simulink model "TCS5"  (R2018b)
settings: Solver=VariableStepAuto  StartTime=0.0  StopTime=10  RelTol=1e-3
model workspace (MAT data in the model file):
  MCOS : class17 (value not decoded)
  MCOS : class17 (value not decoded)
  MCOS : class17 (value not decoded)
  MCOS : class17 (value not decoded)
  MCOS : class17 (value not decoded)
  MCOS : class17 (value not decoded)
undefined symbols (not defined in the file): DiscIntNeverNeededParam
libraries: simulink x8, Solver_SF x1
(part 2 of 2)

== system TCS5/TCS_Control/Axle_3/PID控制器2 ==
  期望驱动力矩 : Inport
  差值 : Inport  Port=2
  Enable : Inport  Port=3
  Abs : Abs
  Add : Sum
  Add1 : Sum
  Constant : Constant  Value=0  OutDataTypeStr=fixdt(1,16,5)
  Constant1 : Constant  Value=T_max
  Constant2 : Constant  Value=Kp
  Constant3 : Constant  Value=Ki
  Constant4 : Constant  Value=0
  Discrete-Time Integrator : DiscreteIntegrator  IntegratorMethod=Integration: Backward Euler  ExternalReset=level  SampleTime=-1  ICPrevOutput=DiscIntNeverNeededParam  ICPrevScaledInput=DiscIntNeverNeededParam
  Logical Operator1 : Logic  Operator=NOT  AllPortsSameDT=off  OutDataTypeStr=boolean
  Multiply : Product  OutDataTypeStr=fixdt(1,32,10)
  Multiply1 : Product  OutDataTypeStr=fixdt(1,32,10)
  Relational Operator : RelationalOperator  Operator===  OutDataTypeStr=boolean  RndMeth=Nearest
  Saturation Dynamic : simulink/Discontinuities/Saturation Dynamic  OutMin=[]  OutMax=[]  OutDataTypeStr=Inherit: Same as second input  OutDataType=fixdt(1, 16)  OutScaling=2^-10  DoSatur=off
  Switch : Switch  Criteria=u2 > Threshold
  Unit Delay : UnitDelay  SampleTime=-1
  △T : Outport  VectorParamsAs1DForOutWhenUnconnected=on
  wires:
  Multiply/1 -> Add/1
  Discrete-Time Integrator/1 -> Add/2
  Enable/1 -> Logical Operator1/1
  Multiply1/1 -> Discrete-Time Integrator/1
  Constant3/1 -> Multiply1/2
  Relational Operator/1 -> Unit Delay/1
  Saturation Dynamic/1 -> Relational Operator/2, △T/1
  Constant2/1 -> Multiply/1
  Unit Delay/1 -> Switch/2
  差值/1 -> Switch/1, Multiply/2
  Add/1 -> Saturation Dynamic/2, Relational Operator/1
  Logical Operator1/1 -> Discrete-Time Integrator/2
  Switch/1 -> Multiply1/1
  Constant/1 -> Switch/3
  Constant1/1 -> Add1/1
  Add1/1 -> Saturation Dynamic/1
  期望驱动力矩/1 -> Abs/1
  Abs/1 -> Add1/2
  Constant4/1 -> Saturation Dynamic/3

== system TCS5/TCS_Control/Axle_3/滑转率计算1 ==
  车轮转速 : Inport
  车速 : Inport  Port=2
  Abs : Abs
  Add : Sum  Inputs=+-
  Add1 : Sum
  Constant : Constant  Value=0.001
  Divide : Product  Inputs=*/
  Gain : Gain  Gain=1/3.6
  Gain2 : Gain  Gain=pi/30
  Product : Product
  Saturation : Saturate  UpperLimit=1  LowerLimit=-1
  轮胎滚动半径 : Constant  Value=r
  左轮滑转率 : Outport  VectorParamsAs1DForOutWhenUnconnected=on
  wires:
  Saturation/1 -> 左轮滑转率/1
  Divide/1 -> Saturation/1
  轮胎滚动半径/1 -> Product/2
  Add/1 -> Divide/1
  Product/1 -> Abs/1, Add/1
  车速/1 -> Gain/1
  Gain/1 -> Add/2
  Gain2/1 -> Product/1
  车轮转速/1 -> Gain2/1
  Add1/1 -> Divide/2
  Constant/1 -> Add1/2
  Abs/1 -> Add1/1

== system TCS5/TCS_Control/Axle_3/滑转率计算2 ==
  车轮转速 : Inport
  车速 : Inport  Port=2
  Abs : Abs
  Add : Sum  Inputs=+-
  Add1 : Sum
  Constant : Constant  Value=0.001
  Divide : Product  Inputs=*/
  Gain : Gain  Gain=1/3.6
  Gain2 : Gain  Gain=pi/30
  Product : Product
  Saturation : Saturate  UpperLimit=1  LowerLimit=-1
  轮胎滚动半径 : Constant  Value=r
  右轮滑转率 : Outport  VectorParamsAs1DForOutWhenUnconnected=on
  wires:
  Saturation/1 -> 右轮滑转率/1
  Divide/1 -> Saturation/1
  轮胎滚动半径/1 -> Product/2
  Add/1 -> Divide/1
  Product/1 -> Abs/1, Add/1
  车速/1 -> Gain/1
  Gain/1 -> Add/2
  Gain2/1 -> Product/1
  车轮转速/1 -> Gain2/1
  Add1/1 -> Divide/2
  Constant/1 -> Add1/2
  Abs/1 -> Add1/1

== system TCS5/TCS_Control/Axle_5/PID控制器1 ==
  期望驱动力矩 : Inport
  差值 : Inport  Port=2
  Enable : Inport  Port=3
  Abs : Abs
  Add : Sum
  Add1 : Sum
  Constant : Constant  Value=0  OutDataTypeStr=fixdt(1,16,5)
  Constant1 : Constant  Value=T_max
  Constant2 : Constant  Value=Kp
  Constant3 : Constant  Value=Ki
  Constant4 : Constant  Value=0
  Discrete-Time Integrator : DiscreteIntegrator  IntegratorMethod=Integration: Backward Euler  ExternalReset=level  SampleTime=-1  ICPrevOutput=DiscIntNeverNeededParam  ICPrevScaledInput=DiscIntNeverNeededParam
  Logical Operator1 : Logic  Operator=NOT  AllPortsSameDT=off  OutDataTypeStr=boolean
  Multiply : Product  OutDataTypeStr=fixdt(1,32,10)
  Multiply1 : Product  OutDataTypeStr=fixdt(1,32,10)
  Relational Operator : RelationalOperator  Operator===  OutDataTypeStr=boolean  RndMeth=Nearest
  Saturation Dynamic : simulink/Discontinuities/Saturation Dynamic  OutMin=[]  OutMax=[]  OutDataTypeStr=Inherit: Same as second input  OutDataType=fixdt(1, 16)  OutScaling=2^-10  DoSatur=off
  Scope : Scope
  Switch : Switch  Criteria=u2 > Threshold
  Unit Delay : UnitDelay  SampleTime=-1
  △T : Outport  VectorParamsAs1DForOutWhenUnconnected=on
  wires:
  Multiply/1 -> Add/1
  Enable/1 -> Logical Operator1/1
  Multiply1/1 -> Discrete-Time Integrator/1
  Constant3/1 -> Multiply1/2
  Relational Operator/1 -> Unit Delay/1
  Saturation Dynamic/1 -> Relational Operator/2, △T/1
  Constant2/1 -> Multiply/1
  Unit Delay/1 -> Switch/2
  差值/1 -> Switch/1, Multiply/2
  Add/1 -> Saturation Dynamic/2, Relational Operator/1
  Logical Operator1/1 -> Discrete-Time Integrator/2
  Switch/1 -> Multiply1/1
  Constant/1 -> Switch/3
  Constant1/1 -> Add1/1
  Add1/1 -> Saturation Dynamic/1
  期望驱动力矩/1 -> Abs/1
  Abs/1 -> Add1/2
  Constant4/1 -> Saturation Dynamic/3
  Discrete-Time Integrator/1 -> Scope/1, Add/2

== system TCS5/TCS_Control/Axle_5/PID控制器2 ==
  期望驱动力矩 : Inport
  差值 : Inport  Port=2
  Enable : Inport  Port=3
  Abs : Abs
  Add : Sum
  Add1 : Sum
  Constant : Constant  Value=0  OutDataTypeStr=fixdt(1,16,5)
  Constant1 : Constant  Value=T_max
  Constant2 : Constant  Value=Kp
  Constant3 : Constant  Value=Ki
  Constant4 : Constant  Value=0
  Discrete-Time Integrator : DiscreteIntegrator  IntegratorMethod=Integration: Backward Euler  ExternalReset=level  SampleTime=-1  ICPrevOutput=DiscIntNeverNeededParam  ICPrevScaledInput=DiscIntNeverNeededParam
  Logical Operator1 : Logic  Operator=NOT  AllPortsSameDT=off  OutDataTypeStr=boolean
  Multiply : Product  OutDataTypeStr=fixdt(1,32,10)
  Multiply1 : Product  OutDataTypeStr=fixdt(1,32,10)
  Relational Operator : RelationalOperator  Operator===  OutDataTypeStr=boolean  RndMeth=Nearest
  Saturation Dynamic : simulink/Discontinuities/Saturation Dynamic  OutMin=[]  OutMax=[]  OutDataTypeStr=Inherit: Same as second input  OutDataType=fixdt(1, 16)  OutScaling=2^-10  DoSatur=off
  Switch : Switch  Criteria=u2 > Threshold
  Unit Delay : UnitDelay  SampleTime=-1
  △T : Outport  VectorParamsAs1DForOutWhenUnconnected=on
  wires:
  Multiply/1 -> Add/1
  Discrete-Time Integrator/1 -> Add/2
  Enable/1 -> Logical Operator1/1
  Multiply1/1 -> Discrete-Time Integrator/1
  Constant3/1 -> Multiply1/2
  Relational Operator/1 -> Unit Delay/1
  Saturation Dynamic/1 -> Relational Operator/2, △T/1
  Constant2/1 -> Multiply/1
  Unit Delay/1 -> Switch/2
  差值/1 -> Switch/1, Multiply/2
  Add/1 -> Saturation Dynamic/2, Relational Operator/1
  Logical Operator1/1 -> Discrete-Time Integrator/2
  Switch/1 -> Multiply1/1
  Constant/1 -> Switch/3
  Constant1/1 -> Add1/1
  Add1/1 -> Saturation Dynamic/1
  期望驱动力矩/1 -> Abs/1
  Abs/1 -> Add1/2
  Constant4/1 -> Saturation Dynamic/3

== system TCS5/TCS_Control/Axle_5/滑转率计算1 ==
  车轮转速 : Inport
  车速 : Inport  Port=2
  Abs : Abs
  Add : Sum  Inputs=+-
  Add1 : Sum
  Constant : Constant  Value=0.001
  Divide : Product  Inputs=*/
  Gain : Gain  Gain=1/3.6
  Gain2 : Gain  Gain=pi/30
  Product : Product
  Saturation : Saturate  UpperLimit=1  LowerLimit=-1
  轮胎滚动半径 : Constant  Value=r
  左轮滑转率 : Outport  VectorParamsAs1DForOutWhenUnconnected=on
  wires:
  Saturation/1 -> 左轮滑转率/1
  Divide/1 -> Saturation/1
  轮胎滚动半径/1 -> Product/2
  Add/1 -> Divide/1
  Product/1 -> Abs/1, Add/1
  车速/1 -> Gain/1
  Gain/1 -> Add/2
  Gain2/1 -> Product/1
  车轮转速/1 -> Gain2/1
  Add1/1 -> Divide/2
  Constant/1 -> Add1/2
  Abs/1 -> Add1/1

== system TCS5/TCS_Control/Axle_5/滑转率计算2 ==
  车轮转速 : Inport
  车速 : Inport  Port=2
  Abs : Abs
  Add : Sum  Inputs=+-
  Add1 : Sum
  Constant : Constant  Value=0.001
  Divide : Product  Inputs=*/
  Gain : Gain  Gain=1/3.6
  Gain2 : Gain  Gain=pi/30
  Product : Product
  Saturation : Saturate  UpperLimit=1  LowerLimit=-1
  轮胎滚动半径 : Constant  Value=r
  右轮滑转率 : Outport  VectorParamsAs1DForOutWhenUnconnected=on
  wires:
  Saturation/1 -> 右轮滑转率/1
  Divide/1 -> Saturation/1
  轮胎滚动半径/1 -> Product/2
  Add/1 -> Divide/1
  Product/1 -> Abs/1, Add/1
  车速/1 -> Gain/1
  Gain/1 -> Add/2
  Gain2/1 -> Product/1
  车轮转速/1 -> Gain2/1
  Add1/1 -> Divide/2
  Constant/1 -> Add1/2
  Abs/1 -> Add1/1

== stateflow chart TCS5/Subsystem7/换挡逻辑/换档策略  ==
  state P
  state R
  state N
  state D
    state D1
      du:gear=1;
    state D2
      du:gear=2;
    state D3
      du:gear=3;
    state D4
      du:gear=4;
    (default) -> D1
    D1 -> D2 : [v>30]
    D2 -> D3 [order 1] : [v>65]
    D3 -> D4 [order 1] : [v>90]
    D2 -> D1 [order 2] : [v<25]
    D4 -> D3 : [v<85]
    D3 -> D2 [order 2] : [v<60]
  (default) -> P
  P -> (junction 31) : [PP==0]
  R -> (junction 31) : [RR==0]
  (junction 31) -> R [order 2] : [RR==1]
  (junction 31) -> P [order 1] : [PP==1]
  N -> (junction 31) : [RR==0]
  (junction 31) -> D [order 4] : [DD==1]
  D -> (junction 31) : [DD==0]
  (junction 31) -> N [order 3] : [NN==1]
  data: v input; gear output; PP input; RR input; NN input; DD input

== stateflow chart TCS5/Subsystem5/换挡逻辑/换档策略  ==
  state P
  state R
  state N
  state D
    state D1
      du:gear=1;
    state D2
      du:gear=2;
    state D3
      du:gear=3;
    state D4
      du:gear=4;
    (default) -> D1
    D1 -> D2 : [v>30]
    D2 -> D3 [order 1] : [v>65]
    D3 -> D4 [order 1] : [v>90]
    D2 -> D1 [order 2] : [v<25]
    D4 -> D3 : [v<85]
    D3 -> D2 [order 2] : [v<60]
  (default) -> P
  P -> (junction 31) : [PP==0]
  R -> (junction 31) : [RR==0]
  (junction 31) -> R [order 2] : [RR==1]
  (junction 31) -> P [order 1] : [PP==1]
  N -> (junction 31) : [RR==0]
  (junction 31) -> D [order 4] : [DD==1]
  D -> (junction 31) : [DD==0]
  (junction 31) -> N [order 3] : [NN==1]
  data: v input; gear output; PP input; RR input; NN input; DD input

== stateflow chart TCS5/Subsystem6/换挡逻辑/换档策略  ==
  state P
  state R
  state N
  state D
    state D1
      du:gear=1;
    state D2
      du:gear=2;
    state D3
      du:gear=3;
    state D4
      du:gear=4;
    (default) -> D1
    D1 -> D2 : [v>30]
    D2 -> D3 [order 1] : [v>65]
    D3 -> D4 [order 1] : [v>90]
    D2 -> D1 [order 2] : [v<25]
    D4 -> D3 : [v<85]
    D3 -> D2 [order 2] : [v<60]
  (default) -> P
  P -> (junction 31) : [PP==0]
  R -> (junction 31) : [RR==0]
  (junction 31) -> R [order 2] : [RR==1]
  (junction 31) -> P [order 1] : [PP==1]
  N -> (junction 31) : [RR==0]
  (junction 31) -> D [order 4] : [DD==1]
  D -> (junction 31) : [DD==0]
  (junction 31) -> N [order 3] : [NN==1]
  data: v input; gear output; PP input; RR input; NN input; DD input

== stateflow chart TCS5/Subsystem/换挡逻辑/换档策略  ==
  state P
  state R
  state N
  state D
    state D1
      du:gear=1;
    state D2
      du:gear=2;
    state D3
      du:gear=3;
    state D4
      du:gear=4;
    (default) -> D1
    D1 -> D2 : [v>30]
    D2 -> D3 [order 1] : [v>65]
    D3 -> D4 [order 1] : [v>90]
    D2 -> D1 [order 2] : [v<25]
    D4 -> D3 : [v<85]
    D3 -> D2 [order 2] : [v<60]
  (default) -> P
  P -> (junction 31) : [PP==0]
  R -> (junction 31) : [RR==0]
  (junction 31) -> R [order 2] : [RR==1]
  (junction 31) -> P [order 1] : [PP==1]
  N -> (junction 31) : [RR==0]
  (junction 31) -> D [order 4] : [DD==1]
  D -> (junction 31) : [DD==0]
  (junction 31) -> N [order 3] : [NN==1]
  data: v input; gear output; PP input; RR input; NN input; DD input

== stateflow chart TCS5/Subsystem1/换挡逻辑/换档策略  ==
  state P
  state R
  state N
  state D
    state D1
      du:gear=1;
    state D2
      du:gear=2;
    state D3
      du:gear=3;
    state D4
      du:gear=4;
    (default) -> D1
    D1 -> D2 : [v>30]
    D2 -> D3 [order 1] : [v>65]
    D3 -> D4 [order 1] : [v>90]
    D2 -> D1 [order 2] : [v<25]
    D4 -> D3 : [v<85]
    D3 -> D2 [order 2] : [v<60]
  (default) -> P
  P -> (junction 31) : [PP==0]
  R -> (junction 31) : [RR==0]
  (junction 31) -> R [order 2] : [RR==1]
  (junction 31) -> P [order 1] : [PP==1]
  N -> (junction 31) : [RR==0]
  (junction 31) -> D [order 4] : [DD==1]
  D -> (junction 31) : [DD==0]
  (junction 31) -> N [order 3] : [NN==1]
  data: v input; gear output; PP input; RR input; NN input; DD input
